simulink model "exsim6_ss_model"  (R2018b)
settings: Solver=VariableStepAuto  StartTime=0.0  StopTime=10.0  FixedStep=Ts  RelTol=1e-3
values from neighbouring files (symbols this model uses):
  A = [0 1; 0.16 -1]    [exsim6.m]
  B = [0 1]'    [exsim6.m]
  C = [1 0]    [exsim6.m]
  nF = double(linsolve(m,v)')    [exsim6.m]
  Ts = 1    [exsim6.m]
settings Model: Creator=rafael  LastModifiedBy=rafael

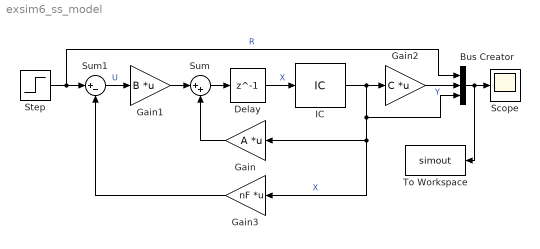
== system exsim6_ss_model ==
  Bus Creator : BusCreator  Inputs=3
  Delay : Delay  DelayLength=1
  Gain : Gain  Gain=A  Multiplication=Matrix(K*u)
  Gain1 : Gain  Gain=B  Multiplication=Matrix(K*u)
  Gain2 : Gain  Gain=C  Multiplication=Matrix(K*u)
  Gain3 : Gain  Gain=nF  Multiplication=Matrix(K*u)
  IC : InitialCondition  Value=[1 -1].^(Ts)
  Scope : Scope
  Step : Step  SampleTime=0
  Sum : Sum  Inputs=|++
  Sum1 : Sum  Inputs=|+-
  To Workspace : ToWorkspace  VariableName=simout  SaveFormat=Timeseries  SampleTime=-1
  wires:
  Sum/1 -> Delay/1
  Gain/1 -> Sum/2
  Gain1/1 -> Sum/1
  Delay/1 -> IC/1  "X"
  Gain3/1 -> Sum1/2
  Sum1/1 -> Gain1/1  "U"
  IC/1 -> Gain/1, Gain3/1, Bus Creator/3, Gain2/1  "X"
  Step/1 -> Bus Creator/1, Sum1/1  "R"
  Bus Creator/1 -> To Workspace/1, Scope/1
  Gain2/1 -> Bus Creator/2  "Y"
